simulink model "simulari"  (R2023b)
settings: Solver=VariableStepAuto  StartTime=0.0  StopTime=400  RelTol=1e-3
undefined symbols (not defined in the file or in its folder): den_PID_chr1_a, den_tangenta, num_PID_chr1_a, num_tangenta
settings Model: Creator=raluc  LastModifiedBy=raluc

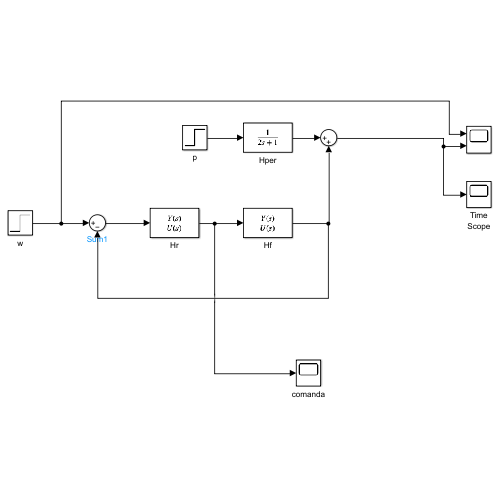
[thumbnail: Simulink's stored preview of the top-level diagram]
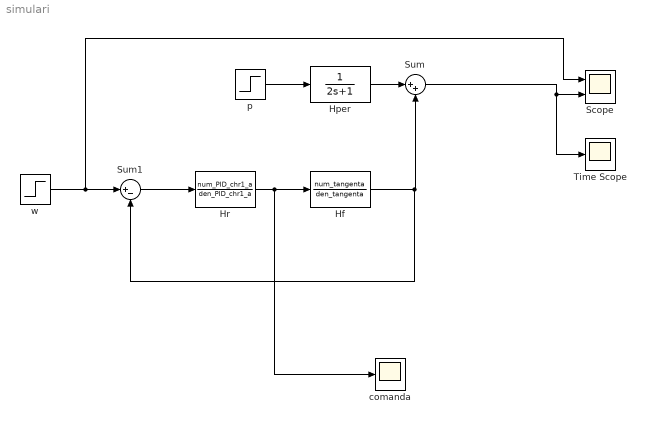
== system simulari ==
  Hf : TransferFcn  Numerator=num_tangenta  Denominator=den_tangenta
  Hper : TransferFcn  Denominator=[2 1]
  Hr : TransferFcn  Numerator=num_PID_chr1_a  Denominator=den_PID_chr1_a
  Scope : Scope  NumInputPorts=2
  Sum : Sum  Inputs=|++
  Sum1 : Sum  Inputs=|+-
  Time Scope : Scope
  comanda : Scope
  p : Step  After=0  SampleTime=0
  w : Step  Time=0  SampleTime=0
  wires:
  Hr/1 -> comanda/1, Hf/1
  Sum/1 -> Time Scope/1, Scope/2
  Hf/1 -> Sum1/2, Sum/2
  Sum1/1 -> Hr/1
  p/1 -> Hper/1
  Hper/1 -> Sum/1
  w/1 -> Sum1/1, Scope/1
